simulink model "PBMRAC_Tuning_Model"  (R2024a)
settings: Solver=VariableStepAuto  StartTime=0.0  StopTime=10.0  RelTol=1e-3
undefined symbols (not defined in the file): a_e_tilde, A_p, B_p, B_pT, Gamma_a, K_p, K_v, L, Lambda_tilde, omega_a_hat_0, p_i_0, R_turn_H, R_turn_V, v_i_0, x_hat_0
libraries: matrix_library x1
settings Model: Creator=Usuario  LastModifiedBy=Usuario

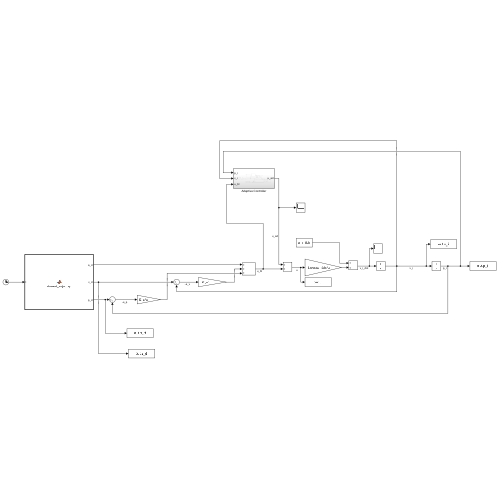
[thumbnail: Simulink's stored preview of the top-level diagram]
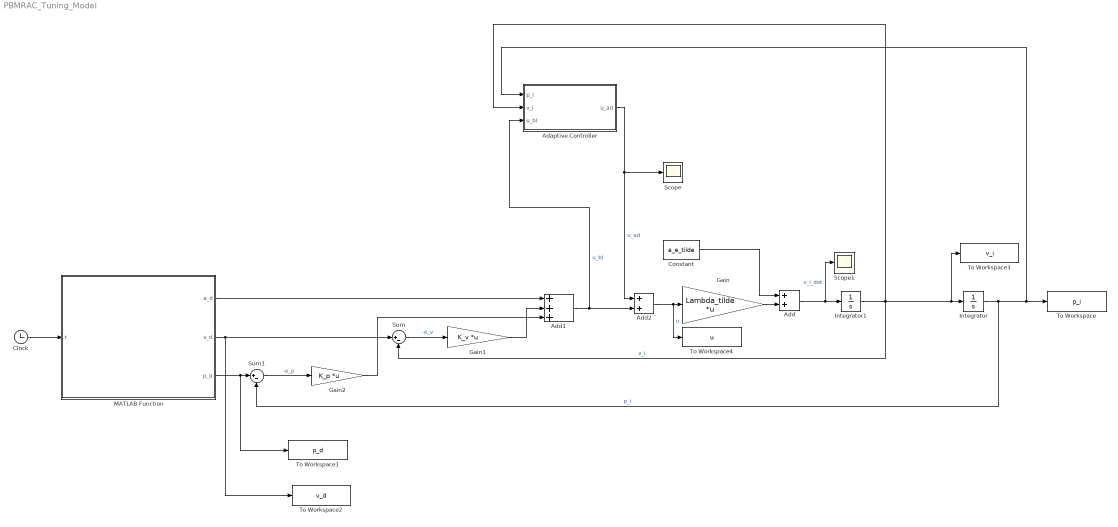
== system PBMRAC_Tuning_Model ==
  Adaptive Controller : Subsystem
  Add : Sum
  Add1 : Sum  Inputs=+++
  Add2 : Sum
  Clock : Clock
  Constant : Constant  Value=a_e_tilde
  Gain : Gain  Gain=Lambda_tilde  Multiplication=Matrix(K*u)
  Gain1 : Gain  Gain=K_v  Multiplication=Matrix(K*u)
  Gain2 : Gain  Gain=K_p  Multiplication=Matrix(K*u)
  Integrator : Integrator  InitialCondition=p_i_0
  Integrator1 : Integrator  InitialCondition=v_i_0
  MATLAB Function : MATLAB Function  TreatAsAtomicUnit=on
  Scope : Scope
  Scope1 : Scope
  Sum : Sum  Inputs=|+-
  Sum1 : Sum  Inputs=|+-
  To Workspace : ToWorkspace  VariableName=p_i  SaveFormat=Timeseries  SampleTime=-1
  To Workspace1 : ToWorkspace  VariableName=p_d  SaveFormat=Timeseries  SampleTime=-1
  To Workspace2 : ToWorkspace  VariableName=v_d  SaveFormat=Timeseries  SampleTime=-1
  To Workspace3 : ToWorkspace  VariableName=v_i  SaveFormat=Timeseries  SampleTime=-1
  To Workspace4 : ToWorkspace  VariableName=u  SaveFormat=Timeseries  SampleTime=-1
  wires:
  Add/1 -> Scope1/1, Integrator1/1  "v_i_dot"
  Integrator1/1 -> Adaptive Controller/2(v_i), To Workspace3/1, Integrator/1, Sum/2  "v_i"
  Integrator/1 -> Adaptive Controller/1(p_i), To Workspace/1, Sum1/2  "p_i"
  Clock/1 -> MATLAB Function/1(t)
  Constant/1 -> Add/1
  Gain/1 -> Add/2
  MATLAB Function/1(a_d) -> Add1/1
  MATLAB Function/2(v_d) -> To Workspace2/1, Sum/1
  MATLAB Function/3(p_d) -> To Workspace1/1, Sum1/1
  Sum/1 -> Gain1/1  "-e_v"
  Sum1/1 -> Gain2/1  "-e_p"
  Gain1/1 -> Add1/2
  Gain2/1 -> Add1/3
  Add1/1 -> Adaptive Controller/3(u_bl), Add2/2  "u_bl"
  Add2/1 -> To Workspace4/1, Gain/1  "u"
  Adaptive Controller/1(u_ad) -> Scope/1, Add2/1  "u_ad"

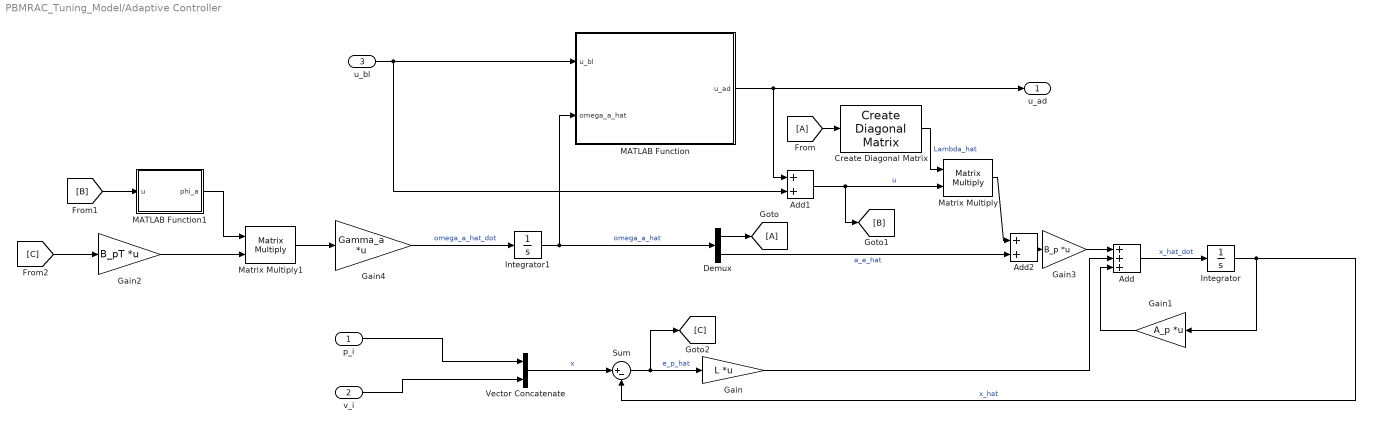
== system PBMRAC_Tuning_Model/Adaptive Controller ==
  p_i : Inport
  v_i : Inport  Port=2
  u_bl : Inport  Port=3
  Add : Sum  Inputs=+++
  Add1 : Sum
  Add2 : Sum
  Create Diagonal Matrix : matrix_library/Create Diagonal Matrix
      settings: LibrarySourceBlock=|
      | simulink/Matrix
      | Operations/Create Diagonal
      | Matrix
  Demux : Demux  Outputs=[3 3]
  From : From
  Gain : Gain  Gain=L  Multiplication=Matrix(K*u)
  Gain1 : Gain  Gain=A_p  Multiplication=Matrix(K*u)
  Gain2 : Gain  Gain=B_pT  Multiplication=Matrix(K*u)
  Gain3 : Gain  Gain=B_p  Multiplication=Matrix(K*u)
  Gain4 : Gain  Gain=Gamma_a  Multiplication=Matrix(K*u)
  Goto : Goto
  Integrator : Integrator  InitialCondition=x_hat_0
  Integrator1 : Integrator  InitialCondition=omega_a_hat_0
  MATLAB Function : MATLAB Function  TreatAsAtomicUnit=on
  MATLAB Function1 : MATLAB Function  TreatAsAtomicUnit=on
  Matrix Multiply : Product  Multiplication=Matrix(*)
  Matrix Multiply1 : Product  Multiplication=Matrix(*)
  Sum : Sum  Inputs=|+-
  Vector Concatenate : Concatenate
  u_ad : Outport
  wires:
  u_bl/1 -> MATLAB Function/1(u_bl), Add1/2
  MATLAB Function/1(u_ad) -> Add1/1, u_ad/1
  Add/1 -> Integrator/1  "x_hat_dot"
  Integrator/1 -> Gain1/1, Sum/2  "x_hat"
  p_i/1 -> Vector Concatenate/1
  v_i/1 -> Vector Concatenate/2
  Vector Concatenate/1 -> Sum/1  "x"
  Sum/1 -> [C], Gain/1  "e_p_hat"
  Gain/1 -> Add/2
  Gain1/1 -> Add/3
  Add2/1 -> Gain3/1
  Add1/1 -> [B], Matrix Multiply/2  "u"
  Create Diagonal Matrix/1 -> Matrix Multiply/1  "Lambda_hat"
  Matrix Multiply/1 -> Add2/1
  Demux/2 -> Add2/2  "a_e_hat"
  Gain4/1 -> Integrator1/1  "omega_a_hat_dot"
  Integrator1/1 -> Demux/1, MATLAB Function/2(omega_a_hat)  "omega_a_hat"
  Demux/1 -> Goto/1
  From/1 -> Create Diagonal Matrix/1
  Matrix Multiply1/1 -> Gain4/1
  [C] -> Gain2/1
  Gain2/1 -> Matrix Multiply1/2
  [B] -> MATLAB Function1/1(u)
  MATLAB Function1/1(phi_a) -> Matrix Multiply1/1
  Gain3/1 -> Add/1

== matlab function PBMRAC_Tuning_Model/Adaptive Controller/MATLAB Function ==
  data: u_bl input; omega_a_hat input; u_ad output
function u_ad=adaptive_control_input(u_bl,omega_a_hat)
Lambda_hat=diag(omega_a_hat(1:3));
a_e_hat=omega_a_hat(4:6);

u_ad=(Lambda_hat\u_bl-u_bl)-Lambda_hat\a_e_hat;
end

== matlab function PBMRAC_Tuning_Model/MATLAB Function ==
  data: a_d output; v_d output; t input; p_d output; R_turn_V parameter; R_turn_H parameter
function [a_d,v_d,p_d]=desired_trajectory(t,R_turn_V, R_turn_H)

[p_d,v_d,a_d,~]=representative_trajectory(t,R_turn_V,R_turn_H);
end

== matlab function PBMRAC_Tuning_Model/Adaptive Controller/MATLAB Function1 ==
  data: u input; phi_a output
function phi_a=construct_phi_a(u)
%This function constructs phi_a for the given augmentation problem. 
phi_a=[diag(u);eye(3,3)];
end
